simulink model "tyre"  (R2017b)
settings: Solver=VariableStepAuto  StartTime=0.0  StopTime=10.0  RelTol=1e-3
settings Model: Creator=Seb  LastModifiedBy=Seb

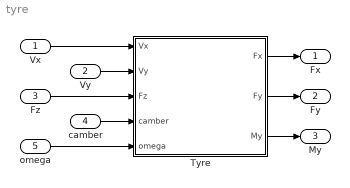
== system tyre ==
  Vx : Inport
  Vy : Inport  Port=2
  Fz : Inport  Port=3
  camber : Inport  Port=4
  omega : Inport  Port=5
  Tyre : Subsystem  mask{TIRFileName="h.tir"}
      mask prompts: TIRFileName "TIR File (String variable)"
      mask Display: image('/Users/Seb/Desktop/tyre.png');
  Fx : Outport
  Fy : Outport  Port=2
  My : Outport  Port=3
  wires:
  Vy/1 -> Tyre/2(Vy)
  omega/1 -> Tyre/5(omega)
  Vx/1 -> Tyre/1(Vx)
  Fz/1 -> Tyre/3(Fz)
  camber/1 -> Tyre/4(camber)
  Tyre/2(Fy) -> Fy/1
  Tyre/3(My) -> My/1
  Tyre/1(Fx) -> Fx/1

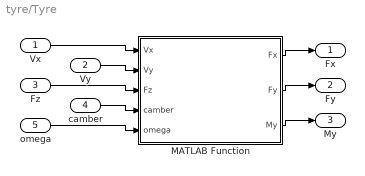
== system tyre/Tyre ==
  Vx : Inport
  Vy : Inport  Port=2
  Fz : Inport  Port=3
  camber : Inport  Port=4
  omega : Inport  Port=5
  MATLAB Function : MATLAB Function  TreatAsAtomicUnit=on
  Fx : Outport
  Fy : Outport  Port=2
  My : Outport  Port=3
  wires:
  camber/1 -> MATLAB Function/4(camber)
  Fz/1 -> MATLAB Function/3(Fz)
  Vy/1 -> MATLAB Function/2(Vy)
  omega/1 -> MATLAB Function/5(omega)
  MATLAB Function/3(My) -> My/1
  MATLAB Function/2(Fy) -> Fy/1
  MATLAB Function/1(Fx) -> Fx/1
  Vx/1 -> MATLAB Function/1(Vx)

== matlab function tyre/Tyre/MATLAB Function ==
  data: Vx input; Fx output; Vy input; Fz input; camber input; omega input; Fy output; My output
function [Fx, Fy, My] = tyre(Vx, Vy, Fz, camber, omega)
Fx =0;
Fy=0;
My = 0;
end
